simulink model "mrefrobotarm_modified_previous_y_previous_u_previous_ref"  (R2018b)
settings: Solver=FixedStepAuto  StartTime=0.0  StopTime=10  RelTol=1e-3  AbsTol=1e-6
undefined symbols (not defined in the file or in its folder): options, sfunxy2
libraries: neural x949, simulink x1
(part 28 of 31)

== system mrefrobotarm_modified_previous_y_previous_u_previous_ref/violates/Layer 1/IW{1,1} ==
  "pd{1,1}" : Inport  PortDimensions=10
      mask Display: e = 0.06;c1 = [120 230 180]/255;c2 = ([120 230 180]+0)/(256+128);c3 = ([120 230 180]+128)/(256+128);patch([0 1 1 0],[0 0 1 1],c1);patch([0 1 1 1-e 1-e 0+e],[0 0 1 1-e 0+e 0+e],c2);patch([0 0 1 1-e 0+e 0+e],[0 1 1 1-e 1-e 0+e],c3);plot([0 1 1 0 0],[0 0 1 1 0]);
  "IW{1,1}(1,:)'" : Constant  Value=[0.8828080088235388256379110316629521548748016357421875;-1.32642130108944744648624691762961447238922119140625;0.260013274525844162443632967551820911467075347900390625;0.38667405203787186263042485734331421554088592529296875;4.2887686070380990344119709334336221218109130859375;-2.364725051554355861327394450199790298938751220703125;-3.20018174030718949296669961768202483654022216796875;0.902716930316901144948360524722374975681304931640625;0.429714323992357538628539259661920368671417236328125;0.1968019529961691216346508781498414464294910430908203125]
      mask Display: e = 0.06;c1 = [120 150 230]/255;c2 = ([120 150 230]+0)/383;c3 = ([120 150 230]+128)/383;patch([0 1 1 0],[0 0 1 1],c1);patch([0 1 1 1-e 1-e 0+e],[0 0 1 1-e 0+e 0+e],c2);patch([0 0 1 1-e 0+e 0+e],[0 1 1 1-e 1-e 0+e],c3);plot([0 1 1 0 0],[0 0 1 1 0]);disp('Weights');
  "IW{1,1}(10,:)'" : Constant  Value=[-0.08573346612905245744951088227026048116385936737060546875;0.49194138381218532884986416320316493511199951171875;-0.659830033779503111190933850593864917755126953125;-0.109656493100025453912849116022698581218719482421875;2.34436657804714965180892249918542802333831787109375;-3.107698692829544473426039985497482120990753173828125;0.465997501487336818204454402803094126284122467041015625;0.542671518807100738968074438162147998809814453125;-1.62571217926619482341266120783984661102294921875;-1.5060132913954216160590249273809604346752166748046875]
      mask Display: e = 0.06;c1 = [120 150 230]/255;c2 = ([120 150 230]+0)/383;c3 = ([120 150 230]+128)/383;patch([0 1 1 0],[0 0 1 1],c1);patch([0 1 1 1-e 1-e 0+e],[0 0 1 1-e 0+e 0+e],c2);patch([0 0 1 1-e 0+e 0+e],[0 1 1 1-e 1-e 0+e],c3);plot([0 1 1 0 0],[0 0 1 1 0]);disp('Weights');
  "IW{1,1}(11,:)'" : Constant  Value=[0.170701186315769748436110830880352295935153961181640625;0.1085512526230558438822271227763849310576915740966796875;0.207116022935932175830231471991282887756824493408203125;0.1153632331976801317363623411438311450183391571044921875;-2.419529772073140794219625604455359280109405517578125;1.819417503322944273946859539137221872806549072265625;0.58370432823550799650291764919529668986797332763671875;-0.331903071260463200520263171711121685802936553955078125;1.7146593036317103742049994252738542854785919189453125;1.5832871492816036340656182801467366516590118408203125]
      mask Display: e = 0.06;c1 = [120 150 230]/255;c2 = ([120 150 230]+0)/383;c3 = ([120 150 230]+128)/383;patch([0 1 1 0],[0 0 1 1],c1);patch([0 1 1 1-e 1-e 0+e],[0 0 1 1-e 0+e 0+e],c2);patch([0 0 1 1-e 0+e 0+e],[0 1 1 1-e 1-e 0+e],c3);plot([0 1 1 0 0],[0 0 1 1 0]);disp('Weights');
  "IW{1,1}(12,:)'" : Constant  Value=[-0.95003585064078299726730847396538592875003814697265625;-0.65738468441400732533708151095197536051273345947265625;0.50911244202974248462822970395791344344615936279296875;0.55946370779339715806344202064792625606060028076171875;4.25736894795902998112069326452910900115966796875;-3.698268745299792659153581553255207836627960205078125;0.82345204855095588403202100380440242588520050048828125;-0.5654120322108895368984349261154420673847198486328125;0.43050272759374619280237084240070544183254241943359375;1.4882266973781728136572155563044361770153045654296875]
      mask Display: e = 0.06;c1 = [120 150 230]/255;c2 = ([120 150 230]+0)/383;c3 = ([120 150 230]+128)/383;patch([0 1 1 0],[0 0 1 1],c1);patch([0 1 1 1-e 1-e 0+e],[0 0 1 1-e 0+e 0+e],c2);patch([0 0 1 1-e 0+e 0+e],[0 1 1 1-e 1-e 0+e],c3);plot([0 1 1 0 0],[0 0 1 1 0]);disp('Weights');
  "IW{1,1}(13,:)'" : Constant  Value=[-0.78775933023882427352901913764071650803089141845703125;1.0334583601767726168674244036083109676837921142578125;2.475745917682078189869798734434880316257476806640625;-1.9403707121873898788777523805038072168827056884765625;0.62955732627357752217989173004752956330776214599609375;-0.2440694773270142559074002974739414639770984649658203125;-1.313726492338394447045857305056415498256683349609375;0.5384731510223497163991623892798088490962982177734375;1.6299218634302885533315929933451116085052490234375;-0.08430793555202431566186760392156429588794708251953125]
      mask Display: e = 0.06;c1 = [120 150 230]/255;c2 = ([120 150 230]+0)/383;c3 = ([120 150 230]+128)/383;patch([0 1 1 0],[0 0 1 1],c1);patch([0 1 1 1-e 1-e 0+e],[0 0 1 1-e 0+e 0+e],c2);patch([0 0 1 1-e 0+e 0+e],[0 1 1 1-e 1-e 0+e],c3);plot([0 1 1 0 0],[0 0 1 1 0]);disp('Weights');
  "IW{1,1}(14,:)'" : Constant  Value=[0.464184773475143586107805049323360435664653778076171875;-0.353787082459256385646995113347657024860382080078125;-0.416992499105133529457845042998087592422962188720703125;0.314956897609315722430523010189062915742397308349609375;-4.18644533231556437158360495232045650482177734375;4.81747291525800758194009176804684102535247802734375;-0.10613141893822665429159002314918325282633304595947265625;-0.363798356601427619327893125955597497522830963134765625;-1.2916791436920547209155074597219936549663543701171875;0.05918663595076741057443570070972782559692859649658203125]
      mask Display: e = 0.06;c1 = [120 150 230]/255;c2 = ([120 150 230]+0)/383;c3 = ([120 150 230]+128)/383;patch([0 1 1 0],[0 0 1 1],c1);patch([0 1 1 1-e 1-e 0+e],[0 0 1 1-e 0+e 0+e],c2);patch([0 0 1 1-e 0+e 0+e],[0 1 1 1-e 1-e 0+e],c3);plot([0 1 1 0 0],[0 0 1 1 0]);disp('Weights');
  "IW{1,1}(15,:)'" : Constant  Value=[0.506356853085071723086230122135020792484283447265625;-1.964538394944709498446400175453163683414459228515625;0.26013577574260005054185285189305432140827178955078125;0.71876470565064654039133529295213520526885986328125;4.82704295385700188347755101858638226985931396484375;-4.07817162644345554411984267062507569789886474609375;-2.1376598360368763707128891837783157825469970703125;1.32077126027228874960428584017790853977203369140625;1.9488054373476746405913218040950596332550048828125;-0.413155719212026595332787337611080147325992584228515625]
      mask Display: e = 0.06;c1 = [120 150 230]/255;c2 = ([120 150 230]+0)/383;c3 = ([120 150 230]+128)/383;patch([0 1 1 0],[0 0 1 1],c1);patch([0 1 1 1-e 1-e 0+e],[0 0 1 1-e 0+e 0+e],c2);patch([0 0 1 1-e 0+e 0+e],[0 1 1 1-e 1-e 0+e],c3);plot([0 1 1 0 0],[0 0 1 1 0]);disp('Weights');
  "IW{1,1}(16,:)'" : Constant  Value=[0.6706245520433398166204597146133892238140106201171875;-0.969425849744247170036715033347718417644500732421875;0.1743449253503210893967434458318166434764862060546875;0.4232811026098775020187758855172432959079742431640625;-5.13832939771205854384561462211422622203826904296875;5.07154158866191107080112487892620265483856201171875;0.06999684391272194272648476953690988011658191680908203125;-0.56459944105790416113421770205604843795299530029296875;0.94022087210700266979301886749453842639923095703125;0.1466554701072172173237362358122481964528560638427734375]
      mask Display: e = 0.06;c1 = [120 150 230]/255;c2 = ([120 150 230]+0)/383;c3 = ([120 150 230]+128)/383;patch([0 1 1 0],[0 0 1 1],c1);patch([0 1 1 1-e 1-e 0+e],[0 0 1 1-e 0+e 0+e],c2);patch([0 0 1 1-e 0+e 0+e],[0 1 1 1-e 1-e 0+e],c3);plot([0 1 1 0 0],[0 0 1 1 0]);disp('Weights');
  "IW{1,1}(17,:)'" : Constant  Value=[1.2401584720564320374336375607526861131191253662109375;0.60746074637946356755691112994099967181682586669921875;-1.485525104640105009679018621682189404964447021484375;0.332463151812849522226400722502148710191249847412109375;-0.7151927336494594555915682576596736907958984375;-1.013651234950070811891009725513868033885955810546875;2.080017416668030083570783972390927374362945556640625;-0.1977189213878693119230689489995711483061313629150390625;-1.6161194659324855660287312275613658130168914794921875;-1.1111159844682265696036438384908251464366912841796875]
      mask Display: e = 0.06;c1 = [120 150 230]/255;c2 = ([120 150 230]+0)/383;c3 = ([120 150 230]+128)/383;patch([0 1 1 0],[0 0 1 1],c1);patch([0 1 1 1-e 1-e 0+e],[0 0 1 1-e 0+e 0+e],c2);patch([0 0 1 1-e 0+e 0+e],[0 1 1 1-e 1-e 0+e],c3);plot([0 1 1 0 0],[0 0 1 1 0]);disp('Weights');
  "IW{1,1}(18,:)'" : Constant  Value=[0.00628639997463334258831491041519257123582065105438232421875;-0.361421779280811150680818855107645504176616668701171875;0.16082768334599906179249728666036389768123626708984375;1.0886234844812106015154995475313626229763031005859375;1.32483882835771549224546106415800750255584716796875;0.2373972048331105810792251986640621908009052276611328125;-1.8529153642295208559431785033666528761386871337890625;0.10892601482705439874809627553986501879990100860595703125;1.3133186886377681279469697983586229383945465087890625;1.242474424853792225320603392901830375194549560546875]
      mask Display: e = 0.06;c1 = [120 150 230]/255;c2 = ([120 150 230]+0)/383;c3 = ([120 150 230]+128)/383;patch([0 1 1 0],[0 0 1 1],c1);patch([0 1 1 1-e 1-e 0+e],[0 0 1 1-e 0+e 0+e],c2);patch([0 0 1 1-e 0+e 0+e],[0 1 1 1-e 1-e 0+e],c3);plot([0 1 1 0 0],[0 0 1 1 0]);disp('Weights');
  "IW{1,1}(19,:)'" : Constant  Value=[-0.7663424268863641142246478921151719987392425537109375;1.982173082691699672608365290216170251369476318359375;-1.098561707938276565954538455116562545299530029296875;-0.128517292366113144996830897071049548685550689697265625;1.75575163364501829477148930891416966915130615234375;-2.172507228415033520008137202239595353603363037109375;0.1994922061979624017258316825973452068865299224853515625;0.319280978911835600086988051771186292171478271484375;-1.029864902578850216485761848161928355693817138671875;-1.13522889484104982926737648085691034793853759765625]
      mask Display: e = 0.06;c1 = [120 150 230]/255;c2 = ([120 150 230]+0)/383;c3 = ([120 150 230]+128)/383;patch([0 1 1 0],[0 0 1 1],c1);patch([0 1 1 1-e 1-e 0+e],[0 0 1 1-e 0+e 0+e],c2);patch([0 0 1 1-e 0+e 0+e],[0 1 1 1-e 1-e 0+e],c3);plot([0 1 1 0 0],[0 0 1 1 0]);disp('Weights');
  "IW{1,1}(2,:)'" : Constant  Value=[-3.599373844422504742368573715793900191783905029296875;5.20790769105741357947181313647888600826263427734375;-5.7085915738761539017787072225473821163177490234375;1.065129691216065932479750699712894856929779052734375;-1.76788717512653992258719881647266447544097900390625;0.893707017671099723798988634371198713779449462890625;0.75065973715547873457154537391033954918384552001953125;1.0508575428428186260276788743794895708560943603515625;-2.1750504167243374098461572430096566677093505859375;-0.463275632999226416597338129577110521495342254638671875]
      mask Display: e = 0.06;c1 = [120 150 230]/255;c2 = ([120 150 230]+0)/383;c3 = ([120 150 230]+128)/383;patch([0 1 1 0],[0 0 1 1],c1);patch([0 1 1 1-e 1-e 0+e],[0 0 1 1-e 0+e 0+e],c2);patch([0 0 1 1-e 0+e 0+e],[0 1 1 1-e 1-e 0+e],c3);plot([0 1 1 0 0],[0 0 1 1 0]);disp('Weights');
  "IW{1,1}(20,:)'" : Constant  Value=[1.5268824929691946490351028842269442975521087646484375;-1.67987268649056620262172145885415375232696533203125;1.987425185489474444011648301966488361358642578125;-1.026589125087584708495569429942406713962554931640625;-1.9819127303341534940273049869574606418609619140625;0.7759508290540237940291490303934551775455474853515625;-0.622016064343394514679630447062663733959197998046875;0.94638566226917741897040059484425000846385955810546875;-1.495419139070976566330273271887563169002532958984375;-2.572866590838346123604196691303513944149017333984375]
      mask Display: e = 0.06;c1 = [120 150 230]/255;c2 = ([120 150 230]+0)/383;c3 = ([120 150 230]+128)/383;patch([0 1 1 0],[0 0 1 1],c1);patch([0 1 1 1-e 1-e 0+e],[0 0 1 1-e 0+e 0+e],c2);patch([0 0 1 1-e 0+e 0+e],[0 1 1 1-e 1-e 0+e],c3);plot([0 1 1 0 0],[0 0 1 1 0]);disp('Weights');
  "IW{1,1}(21,:)'" : Constant  Value=[0.64124071797673642958415030079777352511882781982421875;-1.4222172370065038204955953915487043559551239013671875;1.24718542530506315557659036130644381046295166015625;0.22295568394577569559800167553476057946681976318359375;-4.9690388208638598399602415156550705432891845703125;4.7263369592881900871361722238361835479736328125;-1.7477131936762597685941500458284281194210052490234375;0.857810948082134760994676980772055685520172119140625;-0.50028649944265823901190515243797563016414642333984375;-2.397408489837463019256347251939587295055389404296875]
      mask Display: e = 0.06;c1 = [120 150 230]/255;c2 = ([120 150 230]+0)/383;c3 = ([120 150 230]+128)/383;patch([0 1 1 0],[0 0 1 1],c1);patch([0 1 1 1-e 1-e 0+e],[0 0 1 1-e 0+e 0+e],c2);patch([0 0 1 1-e 0+e 0+e],[0 1 1 1-e 1-e 0+e],c3);plot([0 1 1 0 0],[0 0 1 1 0]);disp('Weights');
  "IW{1,1}(22,:)'" : Constant  Value=[1.3202055555365668215728192080860026180744171142578125;-0.1146805080808551424720320710548548959195613861083984375;-0.080040399876889212205099966013222001492977142333984375;-0.30032731202903872880227709174505434930324554443359375;-5.199913032227453157929630833677947521209716796875;5.8968127505617804473558862810023128986358642578125;-0.8850322746108545413079582431237213313579559326171875;-0.454230335563174436597222438649623654782772064208984375;-2.66920736103003175543335601105354726314544677734375;-1.1179773086774618118255375520675443112850189208984375]
      mask Display: e = 0.06;c1 = [120 150 230]/255;c2 = ([120 150 230]+0)/383;c3 = ([120 150 230]+128)/383;patch([0 1 1 0],[0 0 1 1],c1);patch([0 1 1 1-e 1-e 0+e],[0 0 1 1-e 0+e 0+e],c2);patch([0 0 1 1-e 0+e 0+e],[0 1 1 1-e 1-e 0+e],c3);plot([0 1 1 0 0],[0 0 1 1 0]);disp('Weights');
  "IW{1,1}(23,:)'" : Constant  Value=[-0.74958554116120457155858503028866834938526153564453125;0.3264581040242460208133934429497458040714263916015625;0.5826352141443560395117629013839177787303924560546875;-0.5738309048459895311822265284718014299869537353515625;2.960363743884415921314712250023148953914642333984375;-2.405047008340862380038061019149608910083770751953125;-1.348924529498525703985478685353882610797882080078125;0.8427956295605267822423911638907156884670257568359375;1.1113910978501786441796639337553642690181732177734375;0.25757580721579753646466315331053920090198516845703125]
      mask Display: e = 0.06;c1 = [120 150 230]/255;c2 = ([120 150 230]+0)/383;c3 = ([120 150 230]+128)/383;patch([0 1 1 0],[0 0 1 1],c1);patch([0 1 1 1-e 1-e 0+e],[0 0 1 1-e 0+e 0+e],c2);patch([0 0 1 1-e 0+e 0+e],[0 1 1 1-e 1-e 0+e],c3);plot([0 1 1 0 0],[0 0 1 1 0]);disp('Weights');
  "IW{1,1}(24,:)'" : Constant  Value=[-0.217479751787224728776237725469400174915790557861328125;0.288777756292902976209546750396839343011379241943359375;0.043631879199576041605812548596077249385416507720947265625;-0.2563796600667174185872454472701065242290496826171875;-1.7836885188702893412227012959192506968975067138671875;1.381400295092891195025686101871542632579803466796875;-0.7149435015195118037212296258076094090938568115234375;1.1345687425311086204970933977165259420871734619140625;-0.33911775042697722692963679946842603385448455810546875;0.6594519204924680355617283566971309483051300048828125]
      mask Display: e = 0.06;c1 = [120 150 230]/255;c2 = ([120 150 230]+0)/383;c3 = ([120 150 230]+128)/383;patch([0 1 1 0],[0 0 1 1],c1);patch([0 1 1 1-e 1-e 0+e],[0 0 1 1-e 0+e 0+e],c2);patch([0 0 1 1-e 0+e 0+e],[0 1 1 1-e 1-e 0+e],c3);plot([0 1 1 0 0],[0 0 1 1 0]);disp('Weights');
  "IW{1,1}(25,:)'" : Constant  Value=[-1.307328170367409114760448574088513851165771484375;1.203671529848457044664655768428929150104522705078125;-0.58114212081462734982295614827307872474193572998046875;0.39947922255257062307265414347057230770587921142578125;-3.60541910919981223315744500723667442798614501953125;4.55973331620902211369639189797453582286834716796875;-1.7958019802461568925622259484953247010707855224609375;0.341954122311011132762104125504265539348125457763671875;-2.53228300649411952605305486940778791904449462890625;-1.8285485115086579366305841176654212176799774169921875]
      mask Display: e = 0.06;c1 = [120 150 230]/255;c2 = ([120 150 230]+0)/383;c3 = ([120 150 230]+128)/383;patch([0 1 1 0],[0 0 1 1],c1);patch([0 1 1 1-e 1-e 0+e],[0 0 1 1-e 0+e 0+e],c2);patch([0 0 1 1-e 0+e 0+e],[0 1 1 1-e 1-e 0+e],c3);plot([0 1 1 0 0],[0 0 1 1 0]);disp('Weights');
  "IW{1,1}(26,:)'" : Constant  Value=[0.54706023680647997142756366883986629545688629150390625;-1.5161055461096015761768285301513969898223876953125;1.5021697131739453201504375101649202406406402587890625;-0.003625642823806414678788900829431440797634422779083251953125;-3.065301431948034061036878483719192445278167724609375;3.7182888939074469902834607637487351894378662109375;-0.50283874060600253219632804757566191256046295166015625;-0.387787531069439250774877336880308575928211212158203125;-0.31590750437477110867945384597987867891788482666015625;-0.71838287691313051919195231675985269248485565185546875]
      mask Display: e = 0.06;c1 = [120 150 230]/255;c2 = ([120 150 230]+0)/383;c3 = ([120 150 230]+128)/383;patch([0 1 1 0],[0 0 1 1],c1);patch([0 1 1 1-e 1-e 0+e],[0 0 1 1-e 0+e 0+e],c2);patch([0 0 1 1-e 0+e 0+e],[0 1 1 1-e 1-e 0+e],c3);plot([0 1 1 0 0],[0 0 1 1 0]);disp('Weights');
  "IW{1,1}(27,:)'" : Constant  Value=[0.88132185042763777627072840914479456841945648193359375;-3.360065620633879479584038563189096748828887939453125;1.3887178997527256374411308570415712893009185791015625;0.6302171488579146885200543692917563021183013916015625;6.85431934026103473200919324881397187709808349609375;-5.16599980387182622365571660338900983333587646484375;-1.2286365283502653777958357750321738421916961669921875;0.2002674667992612456135503862242330797016620635986328125;2.76209020535762750370167850633151829242706298828125;2.265467687121908380021295670303516089916229248046875]
      mask Display: e = 0.06;c1 = [120 150 230]/255;c2 = ([120 150 230]+0)/383;c3 = ([120 150 230]+128)/383;patch([0 1 1 0],[0 0 1 1],c1);patch([0 1 1 1-e 1-e 0+e],[0 0 1 1-e 0+e 0+e],c2);patch([0 0 1 1-e 0+e 0+e],[0 1 1 1-e 1-e 0+e],c3);plot([0 1 1 0 0],[0 0 1 1 0]);disp('Weights');
  "IW{1,1}(28,:)'" : Constant  Value=[-0.72339647047768484977581238126731477677822113037109375;0.645162497064734719032230714219622313976287841796875;-0.5714073739005745000696379065630026161670684814453125;0.034450011697239692198824201341267325915396213531494140625;0.470778245531224770470402063438086770474910736083984375;-0.358610121853591146123818589330767281353473663330078125;-0.11762190779038572685522012761794030666351318359375;0.30487188680683841024432467747828923165798187255859375;0.0086927958304470649697481832163248327560722827911376953125;-0.74451387546762959335211462530423887073993682861328125]
      mask Display: e = 0.06;c1 = [120 150 230]/255;c2 = ([120 150 230]+0)/383;c3 = ([120 150 230]+128)/383;patch([0 1 1 0],[0 0 1 1],c1);patch([0 1 1 1-e 1-e 0+e],[0 0 1 1-e 0+e 0+e],c2);patch([0 0 1 1-e 0+e 0+e],[0 1 1 1-e 1-e 0+e],c3);plot([0 1 1 0 0],[0 0 1 1 0]);disp('Weights');
  "IW{1,1}(29,:)'" : Constant  Value=[1.4100244878825112238018846255727112293243408203125;-1.8165250407013122657673420690116472542285919189453125;-0.79505541972619020452128779652412049472332000732421875;0.290852774652112844311346862014033831655979156494140625;0.86368551712939189979323373336228542029857635498046875;-2.766075356327596157512971331016160547733306884765625;1.2605198623439461957929097479791380465030670166015625;1.091779085533283844000607132329605519771575927734375;0.51075425806660390559699180812458507716655731201171875;2.232587803135620330152733004069887101650238037109375]
      mask Display: e = 0.06;c1 = [120 150 230]/255;c2 = ([120 150 230]+0)/383;c3 = ([120 150 230]+128)/383;patch([0 1 1 0],[0 0 1 1],c1);patch([0 1 1 1-e 1-e 0+e],[0 0 1 1-e 0+e 0+e],c2);patch([0 0 1 1-e 0+e 0+e],[0 1 1 1-e 1-e 0+e],c3);plot([0 1 1 0 0],[0 0 1 1 0]);disp('Weights');
  "IW{1,1}(3,:)'" : Constant  Value=[-0.41822920524499174188548522579367272555828094482421875;-0.962862894528984991637798884767107665538787841796875;1.0308931883402154827678032233961857855319976806640625;-0.15150742819952700557450953056104481220245361328125;1.553568049466544920278465724550187587738037109375;-2.40031428028634774562988241086713969707489013671875;0.1326759412630850454295483586975024081766605377197265625;1.0689647434905253930992330424487590789794921875;2.211184265965254081010016307118348777294158935546875;1.4152072954863748055487349120085127651691436767578125]
      mask Display: e = 0.06;c1 = [120 150 230]/255;c2 = ([120 150 230]+0)/383;c3 = ([120 150 230]+128)/383;patch([0 1 1 0],[0 0 1 1],c1);patch([0 1 1 1-e 1-e 0+e],[0 0 1 1-e 0+e 0+e],c2);patch([0 0 1 1-e 0+e 0+e],[0 1 1 1-e 1-e 0+e],c3);plot([0 1 1 0 0],[0 0 1 1 0]);disp('Weights');
  "IW{1,1}(30,:)'" : Constant  Value=[-0.546520993062947990637212569708935916423797607421875;0.14636603855675101026889706190559081733226776123046875;0.0245488184566650217977024084348158794455230236053466796875;0.5627544793248795418350027830456383526325225830078125;0.57691138268121477938876751068164594471454620361328125;-0.0950993246594820373918111044986289925873279571533203125;0.473596798353395576075541839600191451609134674072265625;-0.41062024511850336860874222111306153237819671630859375;-0.755003054329697054214420859352685511112213134765625;0.462692346802911214087572489006561227142810821533203125]
      mask Display: e = 0.06;c1 = [120 150 230]/255;c2 = ([120 150 230]+0)/383;c3 = ([120 150 230]+128)/383;patch([0 1 1 0],[0 0 1 1],c1);patch([0 1 1 1-e 1-e 0+e],[0 0 1 1-e 0+e 0+e],c2);patch([0 0 1 1-e 0+e 0+e],[0 1 1 1-e 1-e 0+e],c3);plot([0 1 1 0 0],[0 0 1 1 0]);disp('Weights');
  "IW{1,1}(4,:)'" : Constant  Value=[1.5913929392104375626360024398309178650379180908203125;-0.91396093254048860199389991976204328238964080810546875;-1.1077312445371363391899421912967227399349212646484375;-0.7995937840342619562505888097803108394145965576171875;2.839729892103999286945281710359267890453338623046875;-1.42261839908866249970742501318454742431640625;-0.08964497308492903882015667704763473011553287506103515625;-0.451786847540717018123501702575595118105411529541015625;1.4254508674080976771136874958756379783153533935546875;-0.12555469342470992888394221154158003628253936767578125]
      mask Display: e = 0.06;c1 = [120 150 230]/255;c2 = ([120 150 230]+0)/383;c3 = ([120 150 230]+128)/383;patch([0 1 1 0],[0 0 1 1],c1);patch([0 1 1 1-e 1-e 0+e],[0 0 1 1-e 0+e 0+e],c2);patch([0 0 1 1-e 0+e 0+e],[0 1 1 1-e 1-e 0+e],c3);plot([0 1 1 0 0],[0 0 1 1 0]);disp('Weights');
  "IW{1,1}(5,:)'" : Constant  Value=[-0.5043632021121846609190697563462890684604644775390625;0.60126738197215623404900952664320357143878936767578125;-0.00621970819720847611922209807744366116821765899658203125;-0.329775071378134609911825236849836073815822601318359375;0.0264223143186110009938971643350669182837009429931640625;0.475828878034194213686447483269148506224155426025390625;0.077129016644802483870790865694289095699787139892578125;-0.095157376028527751454788585760979913175106048583984375;1.6896945456248861905379499148693867027759552001953125;1.186665627041816772901938747963868081569671630859375]
      mask Display: e = 0.06;c1 = [120 150 230]/255;c2 = ([120 150 230]+0)/383;c3 = ([120 150 230]+128)/383;patch([0 1 1 0],[0 0 1 1],c1);patch([0 1 1 1-e 1-e 0+e],[0 0 1 1-e 0+e 0+e],c2);patch([0 0 1 1-e 0+e 0+e],[0 1 1 1-e 1-e 0+e],c3);plot([0 1 1 0 0],[0 0 1 1 0]);disp('Weights');
  "IW{1,1}(6,:)'" : Constant  Value=[-0.652291517640582352299816193408332765102386474609375;2.5408237690908368477948897634632885456085205078125;-1.19703246009394348448040545918047428131103515625;-0.363090723048751173873682773773907683789730072021484375;-5.26523417272079541362472809851169586181640625;4.16082932077967893036429813946597278118133544921875;0.619593638109660727053551454446278512477874755859375;-0.212300769417314960652021227360819466412067413330078125;-1.813237368079999800585255798068828880786895751953125;-1.6119968738863794666116291409707628190517425537109375]
      mask Display: e = 0.06;c1 = [120 150 230]/255;c2 = ([120 150 230]+0)/383;c3 = ([120 150 230]+128)/383;patch([0 1 1 0],[0 0 1 1],c1);patch([0 1 1 1-e 1-e 0+e],[0 0 1 1-e 0+e 0+e],c2);patch([0 0 1 1-e 0+e 0+e],[0 1 1 1-e 1-e 0+e],c3);plot([0 1 1 0 0],[0 0 1 1 0]);disp('Weights');
  "IW{1,1}(7,:)'" : Constant  Value=[1.1733797278533781849318984313867986202239990234375;-2.56849322952456038393620474380441009998321533203125;-0.76450906408746865938752534930245019495487213134765625;0.57154171110927232124510055655264295637607574462890625;-0.0288934685598949934914880799396996735595166683197021484375;1.5388280446938142898005708048003725707530975341796875;-0.76530118230731092321406094924896024167537689208984375;0.5089815860514825818228246134822256863117218017578125;1.9035053061978306487844747607596218585968017578125;0.5900869746271373283974526202655397355556488037109375]
      mask Display: e = 0.06;c1 = [120 150 230]/255;c2 = ([120 150 230]+0)/383;c3 = ([120 150 230]+128)/383;patch([0 1 1 0],[0 0 1 1],c1);patch([0 1 1 1-e 1-e 0+e],[0 0 1 1-e 0+e 0+e],c2);patch([0 0 1 1-e 0+e 0+e],[0 1 1 1-e 1-e 0+e],c3);plot([0 1 1 0 0],[0 0 1 1 0]);disp('Weights');
  "IW{1,1}(8,:)'" : Constant  Value=[1.6314467874675016023644502638489939272403717041015625;-2.391088410740446423830007915967144072055816650390625;0.3491217267537634061369544724584557116031646728515625;0.11565239935715186658793385277022025547921657562255859375;3.49846891837040896433563830214552581310272216796875;-1.5879918072664021000406364692025817930698394775390625;-0.99007253452809973470749582702410407364368438720703125;-0.64122363688064110132103223804733715951442718505859375;1.862589624708915092554661896429024636745452880859375;1.45830711815896396643665866577066481113433837890625]
      mask Display: e = 0.06;c1 = [120 150 230]/255;c2 = ([120 150 230]+0)/383;c3 = ([120 150 230]+128)/383;patch([0 1 1 0],[0 0 1 1],c1);patch([0 1 1 1-e 1-e 0+e],[0 0 1 1-e 0+e 0+e],c2);patch([0 0 1 1-e 0+e 0+e],[0 1 1 1-e 1-e 0+e],c3);plot([0 1 1 0 0],[0 0 1 1 0]);disp('Weights');
  "IW{1,1}(9,:)'" : Constant  Value=[-0.109431419235176463633507637496222741901874542236328125;0.243217577884377866848097937690909020602703094482421875;0.148880442976750348993419947873917408287525177001953125;0.58728154273280963604264570676605217158794403076171875;-4.862587459349100527106202207505702972412109375;4.67000252410542771031032316386699676513671875;0.60699308890144632044894024147652089595794677734375;-0.9186156925029613784516868690843693912029266357421875;-0.8655065020840364553578183404169976711273193359375;0.052826009661363047820170635304748429916799068450927734375]
      mask Display: e = 0.06;c1 = [120 150 230]/255;c2 = ([120 150 230]+0)/383;c3 = ([120 150 230]+128)/383;patch([0 1 1 0],[0 0 1 1],c1);patch([0 1 1 1-e 1-e 0+e],[0 0 1 1-e 0+e 0+e],c2);patch([0 0 1 1-e 0+e 0+e],[0 1 1 1-e 1-e 0+e],c3);plot([0 1 1 0 0],[0 0 1 1 0]);disp('Weights');
  Mux : Mux  Inputs=30
      mask Display: e = 0.06;c1 = [120 150 230]/255;c2 = ([120 150 230]+0)/383;c3 = ([120 150 230]+128)/383;patch([0 1 1 0],[0 0 1 1],c1);patch([0 1 1 1-e 1-e 0+e],[0 0 1 1-e 0+e 0+e],c2);patch([0 0 1 1-e 0+e 0+e],[0 1 1 1-e 1-e 0+e],c3);plot([0 1 1 0 0],[0 0 1 1 0]);disp('Mux');
  dotprod{1..30} (30 alike) : neural/Weight Functions/dotprod
  "iz{1,1}" : Outport
      mask Display: e = 0.06;c1 = [120 230 180]/255;c2 = ([120 230 180]+0)/(256+128);c3 = ([120 230 180]+128)/(256+128);patch([0 1 1 0],[0 0 1 1],c1);patch([0 1 1 1-e 1-e 0+e],[0 0 1 1-e 0+e 0+e],c2);patch([0 0 1 1-e 0+e 0+e],[0 1 1 1-e 1-e 0+e],c3);plot([0 1 1 0 0],[0 0 1 1 0]);
  wires:
  "IW{1,1}(1,:)'"/1 -> dotprod1/1
  "pd{1,1}"/1 -> dotprod1/2, dotprod2/2, dotprod3/2, dotprod4/2, dotprod5/2, dotprod6/2, dotprod7/2, dotprod8/2, dotprod9/2, dotprod10/2, dotprod11/2, dotprod12/2, dotprod13/2, dotprod14/2, dotprod15/2, dotprod16/2, dotprod17/2, dotprod18/2, dotprod19/2, dotprod20/2, dotprod21/2, dotprod22/2, dotprod23/2, dotprod24/2, dotprod25/2, dotprod26/2, dotprod27/2, dotprod28/2, dotprod29/2, dotprod30/2
  dotprod1/1 -> Mux/1
  "IW{1,1}(2,:)'"/1 -> dotprod2/1
  dotprod2/1 -> Mux/2
  "IW{1,1}(3,:)'"/1 -> dotprod3/1
  dotprod3/1 -> Mux/3
  "IW{1,1}(4,:)'"/1 -> dotprod4/1
  dotprod4/1 -> Mux/4
  "IW{1,1}(5,:)'"/1 -> dotprod5/1
  dotprod5/1 -> Mux/5
  "IW{1,1}(6,:)'"/1 -> dotprod6/1
  dotprod6/1 -> Mux/6
  "IW{1,1}(7,:)'"/1 -> dotprod7/1
  dotprod7/1 -> Mux/7
  "IW{1,1}(8,:)'"/1 -> dotprod8/1
  dotprod8/1 -> Mux/8
  "IW{1,1}(9,:)'"/1 -> dotprod9/1
  dotprod9/1 -> Mux/9
  "IW{1,1}(10,:)'"/1 -> dotprod10/1
  dotprod10/1 -> Mux/10
  "IW{1,1}(11,:)'"/1 -> dotprod11/1
  dotprod11/1 -> Mux/11
  "IW{1,1}(12,:)'"/1 -> dotprod12/1
  dotprod12/1 -> Mux/12
  "IW{1,1}(13,:)'"/1 -> dotprod13/1
  dotprod13/1 -> Mux/13
  "IW{1,1}(14,:)'"/1 -> dotprod14/1
  dotprod14/1 -> Mux/14
  "IW{1,1}(15,:)'"/1 -> dotprod15/1
  dotprod15/1 -> Mux/15
  "IW{1,1}(16,:)'"/1 -> dotprod16/1
  dotprod16/1 -> Mux/16
  "IW{1,1}(17,:)'"/1 -> dotprod17/1
  dotprod17/1 -> Mux/17
  "IW{1,1}(18,:)'"/1 -> dotprod18/1
  dotprod18/1 -> Mux/18
  "IW{1,1}(19,:)'"/1 -> dotprod19/1
  dotprod19/1 -> Mux/19
  "IW{1,1}(20,:)'"/1 -> dotprod20/1
  dotprod20/1 -> Mux/20
  "IW{1,1}(21,:)'"/1 -> dotprod21/1
  dotprod21/1 -> Mux/21
  "IW{1,1}(22,:)'"/1 -> dotprod22/1
  dotprod22/1 -> Mux/22
  "IW{1,1}(23,:)'"/1 -> dotprod23/1
  dotprod23/1 -> Mux/23
  "IW{1,1}(24,:)'"/1 -> dotprod24/1
  dotprod24/1 -> Mux/24
  "IW{1,1}(25,:)'"/1 -> dotprod25/1
  dotprod25/1 -> Mux/25
  "IW{1,1}(26,:)'"/1 -> dotprod26/1
  dotprod26/1 -> Mux/26
  "IW{1,1}(27,:)'"/1 -> dotprod27/1
  dotprod27/1 -> Mux/27
  "IW{1,1}(28,:)'"/1 -> dotprod28/1
  dotprod28/1 -> Mux/28
  "IW{1,1}(29,:)'"/1 -> dotprod29/1
  dotprod29/1 -> Mux/29
  "IW{1,1}(30,:)'"/1 -> dotprod30/1
  dotprod30/1 -> Mux/30
  Mux/1 -> "iz{1,1}"/1

== system mrefrobotarm_modified_previous_y_previous_u_previous_ref/violates/Layer 2/Delays 1 ==
  "p{2}" : Inport  PortDimensions=30
      mask Display: e = 0.06;c1 = [120 230 180]/255;c2 = ([120 230 180]+0)/(256+128);c3 = ([120 230 180]+128)/(256+128);patch([0 1 1 0],[0 0 1 1],c1);patch([0 1 1 1-e 1-e 0+e],[0 0 1 1-e 0+e 0+e],c2);patch([0 0 1 1-e 0+e 0+e],[0 1 1 1-e 1-e 0+e],c3);plot([0 1 1 0 0],[0 0 1 1 0]);
  mux : Mux  Inputs=1
      mask Display: e = 0.06;c1 = [120 150 230]/255;c2 = ([120 150 230]+0)/383;c3 = ([120 150 230]+128)/383;patch([0 1 1 0],[0 0 1 1],c1);patch([0 1 1 1-e 1-e 0+e],[0 0 1 1-e 0+e 0+e],c2);patch([0 0 1 1-e 0+e 0+e],[0 1 1 1-e 1-e 0+e],c3);plot([0 1 1 0 0],[0 0 1 1 0]);disp('Mux')
  "pd{2,1}" : Outport
      mask Display: e = 0.06;c1 = [120 230 180]/255;c2 = ([120 230 180]+0)/(256+128);c3 = ([120 230 180]+128)/(256+128);patch([0 1 1 0],[0 0 1 1],c1);patch([0 1 1 1-e 1-e 0+e],[0 0 1 1-e 0+e 0+e],c2);patch([0 0 1 1-e 0+e 0+e],[0 1 1 1-e 1-e 0+e],c3);plot([0 1 1 0 0],[0 0 1 1 0]);
  wires:
  "p{2}"/1 -> mux/1
  mux/1 -> "pd{2,1}"/1
